simulink model "three_phase_bridge_cr"  (Simulink 6.1)
settings: Solver=ode23tb  StartTime=0.0  StopTime=0.1499  MaxStep=1e-4  RelTol=1e-3  AbsTol=.01
libraries: powerlib x16
settings Model: LastModifiedBy=ThinkPad
settings DebuggingCC: SolverPrmCheckMsg=warning

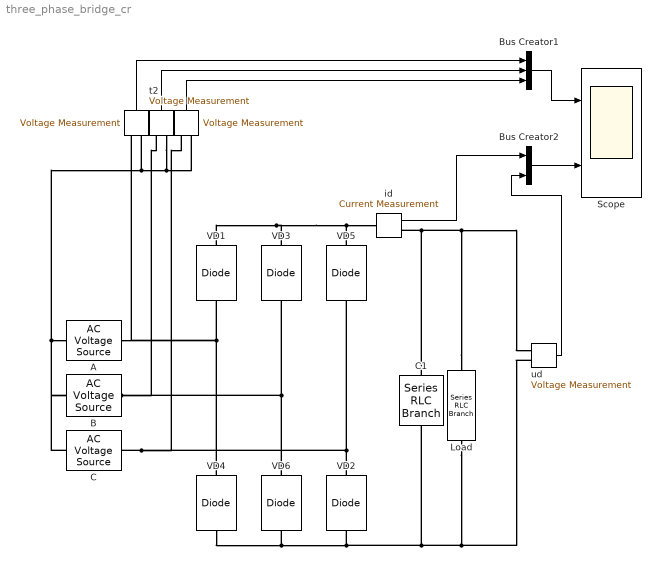
== system three_phase_bridge_cr ==
  " " : powerlib/Measurements/Voltage Measurement  Orientation=up  PhasorSimulation=off  OutputType=Complex  PSBequivalent=0
  "   " : powerlib/Measurements/Voltage Measurement  Orientation=up  PhasorSimulation=off  OutputType=Complex  PSBequivalent=0
  A : powerlib/Electrical Sources/AC Voltage Source  Amplitude=50  Phase=30  Frequency=50  SampleTime=0  Measurements=None
  B : powerlib/Electrical Sources/AC Voltage Source  Amplitude=50  Phase=-90  Frequency=50  SampleTime=0  Measurements=None
  Bus Creator1 : BusCreator  DialogController=Simulink.DDGSource_Bus  Inputs=3
  Bus Creator2 : BusCreator  DialogController=Simulink.DDGSource_Bus  Inputs=2
  C : powerlib/Electrical Sources/AC Voltage Source  Amplitude=50  Phase=-210  Frequency=50  SampleTime=0  Measurements=None
  C1 : powerlib/Elements/Series RLC Branch  Orientation=up  PhysicalDomain=powersysdomain  SubClassName=unknown  LeftPortType=p1  RightPortType=p1  LConnTagsString=__new0  RConnTagsString=__new0  Resistance=0  Inductance=0  Capacitance=0.002  Measurements=None
  Load : powerlib/Elements/Series RLC Branch  Orientation=down  PhysicalDomain=powersysdomain  SubClassName=unknown  LeftPortType=p1  RightPortType=p1  LConnTagsString=__new0  RConnTagsString=__new0  Resistance=5  Inductance=0  Capacitance=inf  Measurements=None
  Scope : Scope  NumInputPorts=2
      settings: TimeRange=0.05  YMin=-50~0  YMax=50~100  Decimation=5  SampleInput=on  SampleTime=1e-4
  VD{1..6} (6 alike) : powerlib/Power Electronics/Diode  Orientation=up  Ron=0.001  Lon=0  Vf=0.8  IC=0  Rs=500  Cs=250e-9  Measurements=off
  id : powerlib/Measurements/Current Measurement  PhasorSimulation=off  OutputType=Complex  PSBequivalent=0
  t2 : powerlib/Measurements/Voltage Measurement  Orientation=up  PhasorSimulation=off  OutputType=Complex  PSBequivalent=0
  ud : powerlib/Measurements/Voltage Measurement  PhasorSimulation=off  OutputType=Complex  PSBequivalent=0
  wires:
  Bus Creator1/1 -> Scope/1
  " "/1 -> Bus Creator1/1
  t2/1 -> Bus Creator1/2
  "   "/1 -> Bus Creator1/3
  Bus Creator2/1 -> Scope/2
  id/1 -> Bus Creator2/1
  ud/1 -> Bus Creator2/2
  connections:
  Load/LConn1 -- ud/LConn1 -- id/RConn1 -- C1/RConn1
  VD5/RConn1 -- VD1/RConn1 -- VD3/RConn1 -- id/LConn1
  C/LConn1 -- B/LConn1 -- A/LConn1 -- t2/LConn2 -- "   "/LConn2 -- " "/LConn2
  VD4/RConn1 -- A/RConn1 -- " "/LConn1 -- VD1/LConn1
  ud/LConn2 -- Load/RConn1 -- VD4/LConn1 -- VD6/LConn1 -- VD2/LConn1 -- C1/LConn1
  VD2/RConn1 -- C/RConn1 -- "   "/LConn1 -- VD5/LConn1
  VD6/RConn1 -- B/RConn1 -- t2/LConn1 -- VD3/LConn1
